simulink model "sampleModel7126_pp_1_1"  (R2018a)
settings: Solver=VariableStepAuto  StartTime=0.0  StopTime=10.0  RelTol=1e-3
undefined symbols (not defined in the file): DiscIntNeverNeededParam
libraries: simulink x367
(part 8 of 12)

== system sampleModel7126_pp_1_1/cfblk263/cfblk3 ==
  emi_1261 : Inport
  emi_1262 : Inport  Port=2
  Action Port : ActionPort  ActionType=then
  cfblk3 : simulink/Continuous/PID Controller (2DOF)  Controller=PID  TimeDomain=Discrete-time  SampleTime=-1  IntegratorMethod=Forward Euler  FilterMethod=Forward Euler  Form=Parallel  UseFilter=on  ControllerParametersSource=internal  P=1  I=1  D=0  N=100  b=1  c=1  InitialConditionSource=internal  InitialConditionForIntegrator=0  InitialConditionForFilter=0  ExternalReset=none  LimitOutput=off  UpperSaturationLimit=inf  LowerSaturationLimit=-inf  LinearizeAsGain=off  AntiWindupMode=none  Kb=1  TrackingMode=off  Kt=1  PParamMin=[]  PParamMax=[]  IParamMin=[]  IParamMax=[]  DParamMin=[]  DParamMax=[]  NParamMin=[]  NParamMax=[]  bParamMin=[]  bParamMax=[]  cParamMin=[]  cParamMax=[]  KbParamMin=[]  KbParamMax=[]  KtParamMin=[]  KtParamMax=[]  POutMin=[]  POutMax=[]  IOutMin=[]  IOutMax=[]  DOutMin=[]  DOutMax=[]  NOutMin=[]  NOutMax=[]  bOutMin=[]  bOutMax=[]  cOutMin=[]  cOutMax=[]  KbOutMin=[]  KbOutMax=[]  KtOutMin=[]  KtOutMax=[]  IntegratorOutMin=[]  IntegratorOutMax=[]  FilterOutMin=[]  FilterOutMax=[]  SumOutMin=[]  SumOutMax=[]  Sum1OutMin=[]  Sum1OutMax=[]  Sum2OutMin=[]  Sum2OutMax=[]  Sum3OutMin=[]  Sum3OutMax=[]  SumI1OutMin=[]  SumI1OutMax=[]  SumI2OutMin=[]  SumI2OutMax=[]  SumI3OutMin=[]  SumI3OutMax=[]  SumDOutMin=[]  SumDOutMax=[]  SaturationOutMin=[]  SaturationOutMax=[]  IntegratorContinuousStateAttributes=''  IntegratorStateMustResolveToSignalObject=off  IntegratorRTWStateStorageClass=Auto  FilterContinuousStateAttributes=''  FilterStateMustResolveToSignalObject=off  FilterRTWStateStorageClass=Auto  DifferentiatorICPrevScaledInput=0  DifferentiatorOutMin=[]  DifferentiatorOutMax=[]  FilterDiffOutCoefMin=[]  FilterDiffOutCoefMax=[]  SumDenOutMin=[]  SumDenOutMax=[]  SumNumOutMin=[]  SumNumOutMax=[]  ReciprocalOutMin=[]  ReciprocalOutMax=[]  DivideOutMin=[]  DivideOutMax=[]  TunerSelectOption=Transfer Function Based (PID Tuner App)
  emi_1263 : Outport
  wires:
  emi_1261/1 -> cfblk3/1
  emi_1262/1 -> cfblk3/2
  cfblk3/1 -> emi_1263/1

== system sampleModel7126_pp_1_1/cfblk263/cfblk4 ==
  emi_867 : Inport
  Action Port : ActionPort  ActionType=then
  cfblk4 : simulink/Discrete/Transfer Fcn Real Zero  ZeroZ=0.75  ICPrevInput=0.0  DoSatur=off
      settings: SourceProductName=Simulink  SourceProductBaseCode=SL
  emi_868 : Outport
  wires:
  emi_867/1 -> cfblk4/1
  cfblk4/1 -> emi_868/1

== system sampleModel7126_pp_1_1/cfblk263/cfblk8 ==
  emi_145 : Inport
  Action Port : ActionPort  ActionType=then
  cfblk8 : DiscreteFir
  emi_146 : Outport
  wires:
  emi_145/1 -> cfblk8/1
  cfblk8/1 -> emi_146/1

== system sampleModel7126_pp_1_1/cfblk263/cfblk9 ==
  emi_1276 : Inport
  Action Port : ActionPort  ActionType=then
  cfblk9 : DiscreteFir
  emi_1277 : Outport
  wires:
  emi_1276/1 -> cfblk9/1
  cfblk9/1 -> emi_1277/1

== system sampleModel7126_pp_1_1/cfblk263/emi_1264 ==
  Action Port : ActionPort  ActionType=else
  emi_1265 : Assertion

== system sampleModel7126_pp_1_1/cfblk263/emi_1278 ==
  Action Port : ActionPort  ActionType=else
  emi_1279 : Assertion

== system sampleModel7126_pp_1_1/cfblk263/emi_147 ==
  Action Port : ActionPort  ActionType=else
  emi_148 : Assertion

== system sampleModel7126_pp_1_1/cfblk263/emi_869 ==
  Action Port : ActionPort  ActionType=else
  emi_870 : Assertion

== system sampleModel7126_pp_1_1/cfblk264/cfblk10 ==
  emi_415 : Inport
  Action Port : ActionPort  ActionType=then
  cfblk10 : simulink/Discrete/Difference  ICPrevInput=0.0  OutMin=[]  OutMax=[]  OutDataTypeStr=double  OutputDataTypeScalingMode=double  OutDataType=fixdt(1, 16)  OutScaling=2^-10  DoSatur=off
  emi_416 : Outport
  wires:
  emi_415/1 -> cfblk10/1
  cfblk10/1 -> emi_416/1

== system sampleModel7126_pp_1_1/cfblk264/cfblk5 ==
  emi_995 : Inport
  Action Port : ActionPort  ActionType=then
  cfblk5 : DiscreteFir
  emi_996 : Outport
  wires:
  emi_995/1 -> cfblk5/1
  cfblk5/1 -> emi_996/1

== system sampleModel7126_pp_1_1/cfblk264/cfblk7 ==
  emi_230 : Inport
  emi_231 : Inport  Port=2
  Action Port : ActionPort  ActionType=then
  cfblk7 : Delay  DelayLengthSource=Input port
      settings: InputPortMap=u0,p1
  emi_232 : Outport
  wires:
  emi_230/1 -> cfblk7/1
  emi_231/1 -> cfblk7/2
  cfblk7/1 -> emi_232/1

== system sampleModel7126_pp_1_1/cfblk264/cfblk8 ==
  emi_1718 : Inport
  Action Port : ActionPort  ActionType=then
  cfblk8 : DiscreteTransferFcn
  emi_1719 : Outport
  wires:
  emi_1718/1 -> cfblk8/1
  cfblk8/1 -> emi_1719/1

== system sampleModel7126_pp_1_1/cfblk264/cfblk9 ==
  emi_1855 : Inport
  Action Port : ActionPort  ActionType=then
  cfblk9 : simulink/Continuous/PID Controller  Controller=PID  TimeDomain=Discrete-time  SampleTime=-1  IntegratorMethod=Forward Euler  FilterMethod=Forward Euler  Form=Parallel  UseFilter=on  ControllerParametersSource=internal  P=1  I=1  D=0  N=100  InitialConditionSource=internal  InitialConditionForIntegrator=0  InitialConditionForFilter=0  ExternalReset=none  LimitOutput=off  UpperSaturationLimit=inf  LowerSaturationLimit=-inf  LinearizeAsGain=off  AntiWindupMode=none  Kb=1  TrackingMode=off  Kt=1  PParamMin=[]  PParamMax=[]  IParamMin=[]  IParamMax=[]  DParamMin=[]  DParamMax=[]  NParamMin=[]  NParamMax=[]  KbParamMin=[]  KbParamMax=[]  KtParamMin=[]  KtParamMax=[]  POutMin=[]  POutMax=[]  IOutMin=[]  IOutMax=[]  DOutMin=[]  DOutMax=[]  NOutMin=[]  NOutMax=[]  KbOutMin=[]  KbOutMax=[]  KtOutMin=[]  KtOutMax=[]  IntegratorOutMin=[]  IntegratorOutMax=[]  FilterOutMin=[]  FilterOutMax=[]  SumOutMin=[]  SumOutMax=[]  SumI1OutMin=[]  SumI1OutMax=[]  SumI2OutMin=[]  SumI2OutMax=[]  SumI3OutMin=[]  SumI3OutMax=[]  SumDOutMin=[]  SumDOutMax=[]  SaturationOutMin=[]  SaturationOutMax=[]  IntegratorContinuousStateAttributes=''  IntegratorStateMustResolveToSignalObject=off  IntegratorRTWStateStorageClass=Auto  FilterContinuousStateAttributes=''  FilterStateMustResolveToSignalObject=off  FilterRTWStateStorageClass=Auto  DifferentiatorICPrevScaledInput=0  DifferentiatorOutMin=[]  DifferentiatorOutMax=[]  FilterDiffOutCoefMin=[]  FilterDiffOutCoefMax=[]  SumDenOutMin=[]  SumDenOutMax=[]  SumNumOutMin=[]  SumNumOutMax=[]  ReciprocalOutMin=[]  ReciprocalOutMax=[]  DivideOutMin=[]  DivideOutMax=[]  TunerSelectOption=Transfer Function Based (PID Tuner App)
  emi_1856 : Outport
  wires:
  emi_1855/1 -> cfblk9/1
  cfblk9/1 -> emi_1856/1

== system sampleModel7126_pp_1_1/cfblk264/emi_1720 ==
  Action Port : ActionPort  ActionType=else
  emi_1721 : Assertion

== system sampleModel7126_pp_1_1/cfblk264/emi_1857 ==
  Action Port : ActionPort  ActionType=else
  emi_1858 : Assertion

== system sampleModel7126_pp_1_1/cfblk264/emi_233 ==
  Action Port : ActionPort  ActionType=else
  emi_234 : Assertion

== system sampleModel7126_pp_1_1/cfblk264/emi_417 ==
  Action Port : ActionPort  ActionType=else
  emi_418 : Assertion

== system sampleModel7126_pp_1_1/cfblk264/emi_997 ==
  Action Port : ActionPort  ActionType=else
  emi_998 : Assertion

== system sampleModel7126_pp_1_1/cfblk265/cfblk10 ==
  cfblk1 : Inport
  cfblk11 : Inport  Port=2
  cfblk12 : Inport  Port=3
  cfblk13 : Inport  Port=4
  cfblk14 : Inport  Port=5
  Action Port : ActionPort  ActionType=else
  cfblk10 : DiscreteStateSpace  SampleTime=-1
  cfblk3 : Delay
  cfblk4 : DiscreteFir
  cfblk5 : simulink/Discrete/Transfer Fcn Lead or Lag  PoleZ=0.95  ZeroZ=0.75  ICPrevOutput=0.0  ICPrevInput=0.0  DoSatur=off
      settings: SourceProductName=Simulink  SourceProductBaseCode=SL
  cfblk6 : Subsystem  TreatAsAtomicUnit=on
  cfblk7 : DiscreteZeroPole  Poles=[0 0.5]  Gain=1  SampleTime=-1
  cfblk8 : DiscreteZeroPole  Poles=[0 0.5]  Gain=1  SampleTime=-1
  cfblk9 : simulink/Discrete/Difference  ICPrevInput=0.0  OutMin=[]  OutMax=[]  OutDataTypeStr=double  OutputDataTypeScalingMode=double  OutDataType=fixdt(1, 16)  OutScaling=2^-10  DoSatur=off
  cyemi_{554..561} (8 alike) : DataTypeConversion  OutDataTypeStr=double
  emi_933 : Subsystem  TreatAsAtomicUnit=on
  emi_935 : If  IfExpression=0 <= u1  SampleTime=[1 0]
  emi_936 : DataTypeConversion  OutDataTypeStr=double
  cfblk2 : Outport
  cfblk15 : Outport  Port=2
  wires:
  cfblk3/1 -> cfblk15/1
  cfblk11/1 -> cfblk2/1
  cyemi_554/1 -> cfblk10/1
  cfblk13/1 -> cyemi_554/1
  cyemi_555/1 -> cfblk3/1
  cfblk8/1 -> cyemi_555/1
  cyemi_556/1 -> cfblk4/1
  cfblk14/1 -> cyemi_556/1
  cyemi_557/1 -> cfblk5/1
  cfblk4/1 -> cyemi_557/1
  cfblk12/1 -> cyemi_558/1
  cyemi_559/1 -> cfblk7/1
  cfblk1/1 -> cyemi_559/1
  cyemi_560/1 -> cfblk8/1
  cyemi_561/1 -> cfblk9/1
  cfblk7/1 -> cyemi_561/1, emi_936/1
  cyemi_558/1 -> cfblk6/1(emi_931)
  cfblk6/1(emi_932) -> cyemi_560/1
  emi_935/1 -> cfblk6/Action
  emi_935/2 -> emi_933/Action
  emi_936/1 -> emi_935/1

== system sampleModel7126_pp_1_1/cfblk265/cfblk12 ==
  emi_287 : Inport
  Action Port : ActionPort  ActionType=then
  cfblk12 : Delay
  emi_288 : Outport
  wires:
  emi_287/1 -> cfblk12/1
  cfblk12/1 -> emi_288/1

== system sampleModel7126_pp_1_1/cfblk265/cfblk3 ==
  emi_1305 : Inport
  emi_1306 : Inport  Port=2
  Action Port : ActionPort  ActionType=then
  cfblk3 : Delay  DelayLengthSource=Input port
      settings: InputPortMap=u0,p1
  emi_1307 : Outport
  wires:
  emi_1305/1 -> cfblk3/1
  emi_1306/1 -> cfblk3/2
  cfblk3/1 -> emi_1307/1

== system sampleModel7126_pp_1_1/cfblk265/cfblk9 ==
  cfblk1 : Inport
  cfblk10 : Inport  Port=2
  cfblk11 : Inport  Port=3
  Action Port : ActionPort  ActionType=then
  cfblk3 : DiscreteIntegrator  SampleTime=-1  OutDataTypeStr=double  ICPrevOutput=DiscIntNeverNeededParam  ICPrevScaledInput=DiscIntNeverNeededParam
  cfblk4 : simulink/Continuous/PID Controller  Controller=PID  TimeDomain=Discrete-time  SampleTime=-1  IntegratorMethod=Forward Euler  FilterMethod=Forward Euler  Form=Parallel  UseFilter=on  ControllerParametersSource=internal  P=1  I=1  D=0  N=100  InitialConditionSource=internal  InitialConditionForIntegrator=0  InitialConditionForFilter=0  ExternalReset=none  LimitOutput=off  UpperSaturationLimit=inf  LowerSaturationLimit=-inf  LinearizeAsGain=off  AntiWindupMode=none  Kb=1  TrackingMode=off  Kt=1  PParamMin=[]  PParamMax=[]  IParamMin=[]  IParamMax=[]  DParamMin=[]  DParamMax=[]  NParamMin=[]  NParamMax=[]  KbParamMin=[]  KbParamMax=[]  KtParamMin=[]  KtParamMax=[]  POutMin=[]  POutMax=[]  IOutMin=[]  IOutMax=[]  DOutMin=[]  DOutMax=[]  NOutMin=[]  NOutMax=[]  KbOutMin=[]  KbOutMax=[]  KtOutMin=[]  KtOutMax=[]  IntegratorOutMin=[]  IntegratorOutMax=[]  FilterOutMin=[]  FilterOutMax=[]  SumOutMin=[]  SumOutMax=[]  SumI1OutMin=[]  SumI1OutMax=[]  SumI2OutMin=[]  SumI2OutMax=[]  SumI3OutMin=[]  SumI3OutMax=[]  SumDOutMin=[]  SumDOutMax=[]  SaturationOutMin=[]  SaturationOutMax=[]  IntegratorContinuousStateAttributes=''  IntegratorStateMustResolveToSignalObject=off  IntegratorRTWStateStorageClass=Auto  FilterContinuousStateAttributes=''  FilterStateMustResolveToSignalObject=off  FilterRTWStateStorageClass=Auto  DifferentiatorICPrevScaledInput=0  DifferentiatorOutMin=[]  DifferentiatorOutMax=[]  FilterDiffOutCoefMin=[]  FilterDiffOutCoefMax=[]  SumDenOutMin=[]  SumDenOutMax=[]  SumNumOutMin=[]  SumNumOutMax=[]  ReciprocalOutMin=[]  ReciprocalOutMax=[]  DivideOutMin=[]  DivideOutMax=[]  TunerSelectOption=Transfer Function Based (PID Tuner App)
  cfblk5 : simulink/Continuous/PID Controller (2DOF)  Controller=PID  TimeDomain=Discrete-time  SampleTime=-1  IntegratorMethod=Forward Euler  FilterMethod=Forward Euler  Form=Parallel  UseFilter=on  ControllerParametersSource=internal  P=1  I=1  D=0  N=100  b=1  c=1  InitialConditionSource=internal  InitialConditionForIntegrator=0  InitialConditionForFilter=0  ExternalReset=none  LimitOutput=off  UpperSaturationLimit=inf  LowerSaturationLimit=-inf  LinearizeAsGain=off  AntiWindupMode=none  Kb=1  TrackingMode=off  Kt=1  PParamMin=[]  PParamMax=[]  IParamMin=[]  IParamMax=[]  DParamMin=[]  DParamMax=[]  NParamMin=[]  NParamMax=[]  bParamMin=[]  bParamMax=[]  cParamMin=[]  cParamMax=[]  KbParamMin=[]  KbParamMax=[]  KtParamMin=[]  KtParamMax=[]  POutMin=[]  POutMax=[]  IOutMin=[]  IOutMax=[]  DOutMin=[]  DOutMax=[]  NOutMin=[]  NOutMax=[]  bOutMin=[]  bOutMax=[]  cOutMin=[]  cOutMax=[]  KbOutMin=[]  KbOutMax=[]  KtOutMin=[]  KtOutMax=[]  IntegratorOutMin=[]  IntegratorOutMax=[]  FilterOutMin=[]  FilterOutMax=[]  SumOutMin=[]  SumOutMax=[]  Sum1OutMin=[]  Sum1OutMax=[]  Sum2OutMin=[]  Sum2OutMax=[]  Sum3OutMin=[]  Sum3OutMax=[]  SumI1OutMin=[]  SumI1OutMax=[]  SumI2OutMin=[]  SumI2OutMax=[]  SumI3OutMin=[]  SumI3OutMax=[]  SumDOutMin=[]  SumDOutMax=[]  SaturationOutMin=[]  SaturationOutMax=[]  IntegratorContinuousStateAttributes=''  IntegratorStateMustResolveToSignalObject=off  IntegratorRTWStateStorageClass=Auto  FilterContinuousStateAttributes=''  FilterStateMustResolveToSignalObject=off  FilterRTWStateStorageClass=Auto  DifferentiatorICPrevScaledInput=0  DifferentiatorOutMin=[]  DifferentiatorOutMax=[]  FilterDiffOutCoefMin=[]  FilterDiffOutCoefMax=[]  SumDenOutMin=[]  SumDenOutMax=[]  SumNumOutMin=[]  SumNumOutMax=[]  ReciprocalOutMin=[]  ReciprocalOutMax=[]  DivideOutMin=[]  DivideOutMax=[]  TunerSelectOption=Transfer Function Based (PID Tuner App)
  cfblk6 : simulink/Discrete/Transfer Fcn Lead or Lag  PoleZ=0.95  ZeroZ=0.75  ICPrevOutput=0.0  ICPrevInput=0.0  DoSatur=off
      settings: SourceProductName=Simulink  SourceProductBaseCode=SL
  cfblk7 : DiscreteFir
  cfblk8 : DiscreteFir
  cfblk9 : simulink/Continuous/PID Controller (2DOF)  Controller=PID  TimeDomain=Discrete-time  SampleTime=-1  IntegratorMethod=Forward Euler  FilterMethod=Forward Euler  Form=Parallel  UseFilter=on  ControllerParametersSource=internal  P=1  I=1  D=0  N=100  b=1  c=1  InitialConditionSource=internal  InitialConditionForIntegrator=0  InitialConditionForFilter=0  ExternalReset=none  LimitOutput=off  UpperSaturationLimit=inf  LowerSaturationLimit=-inf  LinearizeAsGain=off  AntiWindupMode=none  Kb=1  TrackingMode=off  Kt=1  PParamMin=[]  PParamMax=[]  IParamMin=[]  IParamMax=[]  DParamMin=[]  DParamMax=[]  NParamMin=[]  NParamMax=[]  bParamMin=[]  bParamMax=[]  cParamMin=[]  cParamMax=[]  KbParamMin=[]  KbParamMax=[]  KtParamMin=[]  KtParamMax=[]  POutMin=[]  POutMax=[]  IOutMin=[]  IOutMax=[]  DOutMin=[]  DOutMax=[]  NOutMin=[]  NOutMax=[]  bOutMin=[]  bOutMax=[]  cOutMin=[]  cOutMax=[]  KbOutMin=[]  KbOutMax=[]  KtOutMin=[]  KtOutMax=[]  IntegratorOutMin=[]  IntegratorOutMax=[]  FilterOutMin=[]  FilterOutMax=[]  SumOutMin=[]  SumOutMax=[]  Sum1OutMin=[]  Sum1OutMax=[]  Sum2OutMin=[]  Sum2OutMax=[]  Sum3OutMin=[]  Sum3OutMax=[]  SumI1OutMin=[]  SumI1OutMax=[]  SumI2OutMin=[]  SumI2OutMax=[]  SumI3OutMin=[]  SumI3OutMax=[]  SumDOutMin=[]  SumDOutMax=[]  SaturationOutMin=[]  SaturationOutMax=[]  IntegratorContinuousStateAttributes=''  IntegratorStateMustResolveToSignalObject=off  IntegratorRTWStateStorageClass=Auto  FilterContinuousStateAttributes=''  FilterStateMustResolveToSignalObject=off  FilterRTWStateStorageClass=Auto  DifferentiatorICPrevScaledInput=0  DifferentiatorOutMin=[]  DifferentiatorOutMax=[]  FilterDiffOutCoefMin=[]  FilterDiffOutCoefMax=[]  SumDenOutMin=[]  SumDenOutMax=[]  SumNumOutMin=[]  SumNumOutMax=[]  ReciprocalOutMin=[]  ReciprocalOutMax=[]  DivideOutMin=[]  DivideOutMax=[]  TunerSelectOption=Transfer Function Based (PID Tuner App)
  cyemi_{580..588} (9 alike) : DataTypeConversion  OutDataTypeStr=double
  cfblk2 : Outport
  wires:
  cfblk6/1 -> cfblk2/1
  cyemi_580/1 -> cfblk3/1
  cfblk1/1 -> cyemi_580/1
  cyemi_581/1 -> cfblk4/1
  cfblk9/1 -> cyemi_581/1
  cyemi_582/1 -> cfblk5/1
  cfblk10/1 -> cyemi_582/1
  cyemi_583/1 -> cfblk5/2
  cfblk7/1 -> cyemi_583/1
  cyemi_584/1 -> cfblk6/1
  cfblk5/1 -> cyemi_584/1
  cyemi_585/1 -> cfblk7/1
  cfblk4/1 -> cyemi_585/1
  cyemi_586/1 -> cfblk8/1
  cfblk3/1 -> cyemi_586/1
  cyemi_587/1 -> cfblk9/1
  cfblk8/1 -> cyemi_587/1
  cyemi_588/1 -> cfblk9/2
  cfblk11/1 -> cyemi_588/1

== system sampleModel7126_pp_1_1/cfblk265/emi_1308 ==
  Action Port : ActionPort  ActionType=else
  emi_1309 : Assertion

== system sampleModel7126_pp_1_1/cfblk265/emi_289 ==
  Action Port : ActionPort  ActionType=else
  emi_290 : Assertion

== system sampleModel7126_pp_1_1/cfblk266/cfblk10 ==
  cfblk1 : Inport
  Action Port : ActionPort  ActionType=else
  cfblk3 : Subsystem  TreatAsAtomicUnit=on
  cfblk4 : Subsystem  TreatAsAtomicUnit=on
  cfblk5 : Subsystem  TreatAsAtomicUnit=on
  cfblk6 : simulink/Discrete/Transfer Fcn Lead or Lag  PoleZ=0.95  ZeroZ=0.75  ICPrevOutput=0.0  ICPrevInput=0.0  DoSatur=off
      settings: SourceProductName=Simulink  SourceProductBaseCode=SL
  cfblk8 : Subsystem  TreatAsAtomicUnit=on
  cyemi_{591..597} (7 alike) : DataTypeConversion  OutDataTypeStr=double
  emi_1880 : Subsystem  TreatAsAtomicUnit=on
  emi_1882 : If  IfExpression=0 <= u1  SampleTime=[1 0]
  emi_{271,526,617,1883} (4 alike) : DataTypeConversion  OutDataTypeStr=double
  emi_268 : Subsystem  TreatAsAtomicUnit=on
  emi_270 : If  IfExpression=0 <= u1
  emi_523 : Subsystem  TreatAsAtomicUnit=on
  emi_525 : If  IfExpression=0 <= u1  SampleTime=[1 0]
  emi_614 : Subsystem  TreatAsAtomicUnit=on
  emi_616 : If  IfExpression=0 <= u1  SampleTime=[1 0]
  cfblk2 : Outport
  cfblk7 : Outport  Port=2
  wires:
  cfblk6/1 -> cyemi_591/1, cyemi_594/1
  cfblk1/1 -> cyemi_593/1
  cyemi_596/1 -> cfblk6/1
  cyemi_591/1 -> cfblk3/1(emi_266)
  cfblk3/1(emi_267) -> cyemi_597/1
  emi_270/1 -> cfblk3/Action
  emi_270/2 -> emi_268/Action
  emi_271/1 -> emi_270/1
  cyemi_594/1 -> cfblk5/1(emi_520)
  cyemi_595/1 -> cfblk5/2(emi_521)
  cfblk5/1(emi_522) -> cfblk7/1, cfblk2/1, emi_617/1, emi_1883/1
  emi_525/1 -> cfblk5/Action
  emi_525/2 -> emi_523/Action
  emi_526/1 -> emi_525/1
  cyemi_597/1 -> cfblk8/1(emi_612)
  cfblk8/1(emi_613) -> emi_526/1, emi_271/1, cyemi_592/1
  emi_616/1 -> cfblk8/Action
  emi_616/2 -> emi_614/Action
  emi_617/1 -> emi_616/1
  cyemi_592/1 -> cfblk4/1(emi_1877)
  cyemi_593/1 -> cfblk4/2(emi_1878)
  cfblk4/1(emi_1879) -> cyemi_596/1, cyemi_595/1
  emi_1882/1 -> cfblk4/Action
  emi_1882/2 -> emi_1880/Action
  emi_1883/1 -> emi_1882/1

== system sampleModel7126_pp_1_1/cfblk266/cfblk12 ==
  emi_924 : Inport
  Action Port : ActionPort  ActionType=then
  cfblk12 : Delay
  emi_925 : Outport
  wires:
  emi_924/1 -> cfblk12/1
  cfblk12/1 -> emi_925/1

== system sampleModel7126_pp_1_1/cfblk266/cfblk14 ==
  emi_1224 : Inport
  Action Port : ActionPort  ActionType=then
  cfblk14 : Delay
  emi_1225 : Outport
  wires:
  emi_1224/1 -> cfblk14/1
  cfblk14/1 -> emi_1225/1

== system sampleModel7126_pp_1_1/cfblk266/cfblk3 ==
  emi_1469 : Inport
  Action Port : ActionPort  ActionType=then
  cfblk3 : UnitDelay  SampleTime=-1
  emi_1470 : Outport
  wires:
  emi_1469/1 -> cfblk3/1
  cfblk3/1 -> emi_1470/1

== system sampleModel7126_pp_1_1/cfblk266/cfblk9 ==
  cfblk1 : Inport
  cfblk6 : Inport  Port=2
  cfblk7 : Inport  Port=3
  Action Port : ActionPort  ActionType=then
  cfblk3 : simulink/Discrete/Difference  ICPrevInput=0.0  OutMin=[]  OutMax=[]  OutDataTypeStr=double  OutputDataTypeScalingMode=double  OutDataType=fixdt(1, 16)  OutScaling=2^-10  DoSatur=off
  cfblk4 : simulink/Discrete/Transfer Fcn Lead or Lag  PoleZ=0.95  ZeroZ=0.75  ICPrevOutput=0.0  ICPrevInput=0.0  DoSatur=off
      settings: SourceProductName=Simulink  SourceProductBaseCode=SL
  cfblk5 : DiscreteIntegrator  SampleTime=-1  OutDataTypeStr=double  ICPrevOutput=DiscIntNeverNeededParam  ICPrevScaledInput=DiscIntNeverNeededParam
  cyemi_612 : DataTypeConversion  OutDataTypeStr=double
  cyemi_613 : DataTypeConversion  OutDataTypeStr=double
  cyemi_614 : DataTypeConversion  OutDataTypeStr=double
  cfblk2 : Outport
  cfblk8 : Outport  Port=2
  wires:
  cfblk5/1 -> cfblk8/1
  cfblk3/1 -> cfblk2/1
  cyemi_612/1 -> cfblk3/1
  cfblk7/1 -> cyemi_612/1
  cyemi_613/1 -> cfblk4/1
  cfblk6/1 -> cyemi_613/1
  cyemi_614/1 -> cfblk5/1
  cfblk1/1 -> cyemi_614/1

== system sampleModel7126_pp_1_1/cfblk266/emi_1226 ==
  Action Port : ActionPort  ActionType=else
  emi_1227 : Assertion

== system sampleModel7126_pp_1_1/cfblk266/emi_1471 ==
  Action Port : ActionPort  ActionType=else
  emi_1472 : Assertion

== system sampleModel7126_pp_1_1/cfblk266/emi_926 ==
  Action Port : ActionPort  ActionType=else
  emi_927 : Assertion

== system sampleModel7126_pp_1_1/cfblk267/cfblk10 ==
  emi_2180 : Inport
  Action Port : ActionPort  ActionType=then
  cfblk10 : DiscreteFilter
  emi_2181 : Outport
  wires:
  emi_2180/1 -> cfblk10/1
  cfblk10/1 -> emi_2181/1

== system sampleModel7126_pp_1_1/cfblk267/cfblk11 ==
  emi_245 : Inport
  Action Port : ActionPort  ActionType=then
  cfblk11 : Delay
  emi_246 : Outport
  wires:
  emi_245/1 -> cfblk11/1
  cfblk11/1 -> emi_246/1

== system sampleModel7126_pp_1_1/cfblk267/cfblk3 ==
  emi_528 : Inport
  Action Port : ActionPort  ActionType=then
  cfblk3 : DiscreteFir
  emi_529 : Outport
  wires:
  emi_528/1 -> cfblk3/1
  cfblk3/1 -> emi_529/1

== system sampleModel7126_pp_1_1/cfblk267/cfblk4 ==
  emi_1334 : Inport
  Action Port : ActionPort  ActionType=then
  cfblk4 : UnitDelay  SampleTime=-1
  emi_1335 : Outport
  wires:
  emi_1334/1 -> cfblk4/1
  cfblk4/1 -> emi_1335/1

== system sampleModel7126_pp_1_1/cfblk267/cfblk5 ==
  emi_1298 : Inport
  Action Port : ActionPort  ActionType=then
  cfblk5 : simulink/Continuous/PID Controller  Controller=PID  TimeDomain=Discrete-time  SampleTime=-1  IntegratorMethod=Forward Euler  FilterMethod=Forward Euler  Form=Parallel  UseFilter=on  ControllerParametersSource=internal  P=1  I=1  D=0  N=100  InitialConditionSource=internal  InitialConditionForIntegrator=0  InitialConditionForFilter=0  ExternalReset=none  LimitOutput=off  UpperSaturationLimit=inf  LowerSaturationLimit=-inf  LinearizeAsGain=off  AntiWindupMode=none  Kb=1  TrackingMode=off  Kt=1  PParamMin=[]  PParamMax=[]  IParamMin=[]  IParamMax=[]  DParamMin=[]  DParamMax=[]  NParamMin=[]  NParamMax=[]  KbParamMin=[]  KbParamMax=[]  KtParamMin=[]  KtParamMax=[]  POutMin=[]  POutMax=[]  IOutMin=[]  IOutMax=[]  DOutMin=[]  DOutMax=[]  NOutMin=[]  NOutMax=[]  KbOutMin=[]  KbOutMax=[]  KtOutMin=[]  KtOutMax=[]  IntegratorOutMin=[]  IntegratorOutMax=[]  FilterOutMin=[]  FilterOutMax=[]  SumOutMin=[]  SumOutMax=[]  SumI1OutMin=[]  SumI1OutMax=[]  SumI2OutMin=[]  SumI2OutMax=[]  SumI3OutMin=[]  SumI3OutMax=[]  SumDOutMin=[]  SumDOutMax=[]  SaturationOutMin=[]  SaturationOutMax=[]  IntegratorContinuousStateAttributes=''  IntegratorStateMustResolveToSignalObject=off  IntegratorRTWStateStorageClass=Auto  FilterContinuousStateAttributes=''  FilterStateMustResolveToSignalObject=off  FilterRTWStateStorageClass=Auto  DifferentiatorICPrevScaledInput=0  DifferentiatorOutMin=[]  DifferentiatorOutMax=[]  FilterDiffOutCoefMin=[]  FilterDiffOutCoefMax=[]  SumDenOutMin=[]  SumDenOutMax=[]  SumNumOutMin=[]  SumNumOutMax=[]  ReciprocalOutMin=[]  ReciprocalOutMax=[]  DivideOutMin=[]  DivideOutMax=[]  TunerSelectOption=Transfer Function Based (PID Tuner App)
  emi_1299 : Outport
  wires:
  emi_1298/1 -> cfblk5/1
  cfblk5/1 -> emi_1299/1

== system sampleModel7126_pp_1_1/cfblk267/cfblk7 ==
  emi_960 : Inport
  Action Port : ActionPort  ActionType=then
  cfblk7 : DiscreteStateSpace  SampleTime=-1
  emi_961 : Outport
  wires:
  emi_960/1 -> cfblk7/1
  cfblk7/1 -> emi_961/1

== system sampleModel7126_pp_1_1/cfblk267/cfblk8 ==
  emi_1117 : Inport
  Action Port : ActionPort  ActionType=then
  cfblk8 : DiscreteZeroPole  Poles=[0 0.5]  Gain=1  SampleTime=-1
  emi_1118 : Outport
  wires:
  emi_1117/1 -> cfblk8/1
  cfblk8/1 -> emi_1118/1

== system sampleModel7126_pp_1_1/cfblk267/emi_1119 ==
  Action Port : ActionPort  ActionType=else
  emi_1120 : Assertion

== system sampleModel7126_pp_1_1/cfblk267/emi_1300 ==
  Action Port : ActionPort  ActionType=else
  emi_1301 : Assertion

== system sampleModel7126_pp_1_1/cfblk267/emi_1336 ==
  Action Port : ActionPort  ActionType=else
  emi_1337 : Assertion

== system sampleModel7126_pp_1_1/cfblk267/emi_2182 ==
  Action Port : ActionPort  ActionType=else
  emi_2183 : Assertion

== system sampleModel7126_pp_1_1/cfblk267/emi_247 ==
  Action Port : ActionPort  ActionType=else
  emi_248 : Assertion

== system sampleModel7126_pp_1_1/cfblk267/emi_530 ==
  Action Port : ActionPort  ActionType=else
  emi_531 : Assertion

== system sampleModel7126_pp_1_1/cfblk267/emi_962 ==
  Action Port : ActionPort  ActionType=else
  emi_963 : Assertion

== system sampleModel7126_pp_1_1/cfblk268/cfblk3 ==
  emi_640 : Inport
  Action Port : ActionPort  ActionType=then
  cfblk3 : DiscreteStateSpace  SampleTime=-1
  emi_641 : Outport
  wires:
  emi_640/1 -> cfblk3/1
  cfblk3/1 -> emi_641/1

== system sampleModel7126_pp_1_1/cfblk268/cfblk5 ==
  emi_1689 : Inport
  Action Port : ActionPort  ActionType=then
  cfblk5 : simulink/Discrete/Transfer Fcn Real Zero  ZeroZ=0.75  ICPrevInput=0.0  DoSatur=off
      settings: SourceProductName=Simulink  SourceProductBaseCode=SL
  emi_1690 : Outport
  wires:
  emi_1689/1 -> cfblk5/1
  cfblk5/1 -> emi_1690/1

== system sampleModel7126_pp_1_1/cfblk268/cfblk8 ==
  emi_1562 : Inport
  Action Port : ActionPort  ActionType=then
  cfblk8 : simulink/Discrete/Transfer Fcn Lead or Lag  PoleZ=0.95  ZeroZ=0.75  ICPrevOutput=0.0  ICPrevInput=0.0  DoSatur=off
      settings: SourceProductName=Simulink  SourceProductBaseCode=SL
  emi_1563 : Outport
  wires:
  emi_1562/1 -> cfblk8/1
  cfblk8/1 -> emi_1563/1

== system sampleModel7126_pp_1_1/cfblk268/emi_1564 ==
  Action Port : ActionPort  ActionType=else
  emi_1565 : Assertion

== system sampleModel7126_pp_1_1/cfblk268/emi_1691 ==
  Action Port : ActionPort  ActionType=else
  emi_1692 : Assertion

== system sampleModel7126_pp_1_1/cfblk268/emi_642 ==
  Action Port : ActionPort  ActionType=else
  emi_643 : Assertion

== system sampleModel7126_pp_1_1/cfblk269/cfblk14 ==
  emi_1740 : Inport
  Action Port : ActionPort  ActionType=then
  cfblk14 : Delay
  emi_1741 : Outport
  wires:
  emi_1740/1 -> cfblk14/1
  cfblk14/1 -> emi_1741/1

== system sampleModel7126_pp_1_1/cfblk269/cfblk3 ==
  emi_1777 : Inport
  Action Port : ActionPort  ActionType=then
  cfblk3 : DiscreteIntegrator  SampleTime=-1  OutDataTypeStr=double  ICPrevOutput=DiscIntNeverNeededParam  ICPrevScaledInput=DiscIntNeverNeededParam
  emi_1778 : Outport
  wires:
  emi_1777/1 -> cfblk3/1
  cfblk3/1 -> emi_1778/1

== system sampleModel7126_pp_1_1/cfblk269/cfblk4 ==
  emi_489 : Inport
  emi_490 : Inport  Port=2
  Action Port : ActionPort  ActionType=then
  cfblk4 : Delay  ShowEnablePort=on
      settings: InputPortMap=u0,e6
  emi_491 : Outport
  wires:
  emi_489/1 -> cfblk4/1
  emi_490/1 -> cfblk4/2
  cfblk4/1 -> emi_491/1

== system sampleModel7126_pp_1_1/cfblk269/cfblk8 ==
  cfblk1 : Inport
  cfblk12 : Inport  Port=2
  cfblk13 : Inport  Port=3
  Action Port : ActionPort  ActionType=then
  cfblk10 : Delay  ShowEnablePort=on
      settings: InputPortMap=u0,e6
  cfblk11 : Subsystem  TreatAsAtomicUnit=on
  cfblk15 : Delay
  cfblk3 : simulink/Continuous/PID Controller  Controller=PID  TimeDomain=Discrete-time  SampleTime=-1  IntegratorMethod=Forward Euler  FilterMethod=Forward Euler  Form=Parallel  UseFilter=on  ControllerParametersSource=internal  P=1  I=1  D=0  N=100  InitialConditionSource=internal  InitialConditionForIntegrator=0  InitialConditionForFilter=0  ExternalReset=none  LimitOutput=off  UpperSaturationLimit=inf  LowerSaturationLimit=-inf  LinearizeAsGain=off  AntiWindupMode=none  Kb=1  TrackingMode=off  Kt=1  PParamMin=[]  PParamMax=[]  IParamMin=[]  IParamMax=[]  DParamMin=[]  DParamMax=[]  NParamMin=[]  NParamMax=[]  KbParamMin=[]  KbParamMax=[]  KtParamMin=[]  KtParamMax=[]  POutMin=[]  POutMax=[]  IOutMin=[]  IOutMax=[]  DOutMin=[]  DOutMax=[]  NOutMin=[]  NOutMax=[]  KbOutMin=[]  KbOutMax=[]  KtOutMin=[]  KtOutMax=[]  IntegratorOutMin=[]  IntegratorOutMax=[]  FilterOutMin=[]  FilterOutMax=[]  SumOutMin=[]  SumOutMax=[]  SumI1OutMin=[]  SumI1OutMax=[]  SumI2OutMin=[]  SumI2OutMax=[]  SumI3OutMin=[]  SumI3OutMax=[]  SumDOutMin=[]  SumDOutMax=[]  SaturationOutMin=[]  SaturationOutMax=[]  IntegratorContinuousStateAttributes=''  IntegratorStateMustResolveToSignalObject=off  IntegratorRTWStateStorageClass=Auto  FilterContinuousStateAttributes=''  FilterStateMustResolveToSignalObject=off  FilterRTWStateStorageClass=Auto  DifferentiatorICPrevScaledInput=0  DifferentiatorOutMin=[]  DifferentiatorOutMax=[]  FilterDiffOutCoefMin=[]  FilterDiffOutCoefMax=[]  SumDenOutMin=[]  SumDenOutMax=[]  SumNumOutMin=[]  SumNumOutMax=[]  ReciprocalOutMin=[]  ReciprocalOutMax=[]  DivideOutMin=[]  DivideOutMax=[]  TunerSelectOption=Transfer Function Based (PID Tuner App)
  cfblk4 : UnitDelay  SampleTime=-1
  cfblk5 : DiscreteIntegrator  SampleTime=-1  OutDataTypeStr=double  ICPrevOutput=DiscIntNeverNeededParam  ICPrevScaledInput=DiscIntNeverNeededParam
  cfblk6 : simulink/Discrete/Tapped Delay  vinit=0.0  samptime=-1  NumDelays=1  DelayOrder=Oldest  includeCurrent=off
  cfblk7 : Subsystem  TreatAsAtomicUnit=on
  cfblk8 : DiscreteZeroPole  Poles=[0 0.5]  Gain=1  SampleTime=-1
  cfblk9 : DiscreteStateSpace  SampleTime=-1
  cyemi_{653..663} (11 alike) : DataTypeConversion  OutDataTypeStr=double
  emi_2075 : Subsystem  TreatAsAtomicUnit=on
  emi_2077 : If  IfExpression=Inf <= u1  SampleTime=[1 0]
  emi_2078 : DataTypeConversion  OutDataTypeStr=double
  emi_955 : Subsystem  TreatAsAtomicUnit=on
  emi_957 : If  IfExpression=Inf <= u1  SampleTime=[1 0]
  emi_958 : DataTypeConversion  OutDataTypeStr=double
  cfblk2 : Outport
  cfblk14 : Outport  Port=2
  wires:
  cfblk8/1 -> cfblk14/1, emi_958/1
  cfblk1/1 -> cfblk2/1
  cyemi_653/1 -> cfblk10/1
  cfblk13/1 -> cyemi_653/1
  cyemi_654/1 -> cfblk10/2
  cfblk3/1 -> cyemi_655/1
  cyemi_656/1 -> cfblk15/1
  cfblk5/1 -> cyemi_656/1
  cyemi_657/1 -> cfblk3/1
  cfblk9/1 -> cyemi_657/1
  cyemi_658/1 -> cfblk4/1
  cfblk15/1 -> cyemi_658/1
  cyemi_659/1 -> cfblk5/1
  cfblk4/1 -> cyemi_659/1, emi_2078/1
  cyemi_660/1 -> cfblk6/1
  cfblk12/1 -> cyemi_660/1
  cyemi_662/1 -> cfblk8/1
  cfblk10/1 -> cyemi_662/1
  cyemi_663/1 -> cfblk9/1
  cfblk6/1 -> cyemi_663/1
  cyemi_655/1 -> cfblk11/1(emi_953)
  cfblk11/1(emi_954) -> cyemi_661/1
  emi_957/1 -> cfblk11/Action
  emi_957/2 -> emi_955/Action
  emi_958/1 -> emi_957/1
  cyemi_661/1 -> cfblk7/1(emi_2073)
  cfblk7/1(emi_2074) -> cyemi_654/1
  emi_2077/1 -> cfblk7/Action
  emi_2077/2 -> emi_2075/Action
  emi_2078/1 -> emi_2077/1

== system sampleModel7126_pp_1_1/cfblk269/cfblk9 ==
  cfblk1 : Inport
  cfblk8 : Inport  Port=2
  cfblk9 : Inport  Port=3
  Action Port : ActionPort  ActionType=else
  cfblk3 : DiscreteStateSpace  SampleTime=-1
  cfblk4 : DiscreteFilter
  cfblk5 : Subsystem  TreatAsAtomicUnit=on
  cfblk6 : Subsystem  TreatAsAtomicUnit=on
  cfblk7 : DiscreteStateSpace  SampleTime=-1
  cyemi_{667..672} (6 alike) : DataTypeConversion  OutDataTypeStr=double
  emi_1198 : Subsystem  TreatAsAtomicUnit=on
  emi_1200 : If  IfExpression=Inf <= u1  SampleTime=[1 0]
  emi_1201 : DataTypeConversion  OutDataTypeStr=double
  emi_275 : Subsystem  TreatAsAtomicUnit=on
  emi_277 : If  IfExpression=Inf <= u1  SampleTime=[1 0]
  emi_278 : DataTypeConversion  OutDataTypeStr=double
  cfblk2 : Outport
  cfblk10 : Outport  Port=2
  cfblk11 : Outport  Port=3
  cfblk12 : Outport  Port=4
  cfblk13 : Outport  Port=5
  wires:
  cfblk1/1 -> cyemi_668/1, cyemi_669/1
  cfblk3/1 -> cfblk10/1, cyemi_670/1, emi_1201/1
  cfblk9/1 -> cfblk13/1
  cfblk4/1 -> cfblk11/1, cyemi_667/1
  cfblk7/1 -> cfblk2/1, emi_278/1
  cyemi_667/1 -> cfblk3/1
  cyemi_668/1 -> cfblk4/1
  cyemi_672/1 -> cfblk7/1
  cfblk8/1 -> cyemi_672/1
  cyemi_671/1 -> cfblk6/1(emi_273)
  cfblk6/1(emi_274) -> cfblk12/1
  emi_277/1 -> cfblk6/Action
  emi_277/2 -> emi_275/Action
  emi_278/1 -> emi_277/1
  cyemi_669/1 -> cfblk5/1(emi_1195)
  cyemi_670/1 -> cfblk5/2(emi_1196)
  cfblk5/1(emi_1197) -> cyemi_671/1
  emi_1200/1 -> cfblk5/Action
  emi_1200/2 -> emi_1198/Action
  emi_1201/1 -> emi_1200/1

== system sampleModel7126_pp_1_1/cfblk269/emi_1742 ==
  Action Port : ActionPort  ActionType=else
  emi_1743 : Assertion

== system sampleModel7126_pp_1_1/cfblk269/emi_1779 ==
  Action Port : ActionPort  ActionType=else
  emi_1780 : Assertion

== system sampleModel7126_pp_1_1/cfblk269/emi_492 ==
  Action Port : ActionPort  ActionType=else
  emi_493 : Assertion

== system sampleModel7126_pp_1_1/cfblk270/cfblk11 ==
  emi_2045 : Inport
  Action Port : ActionPort  ActionType=then
  cfblk11 : Delay
  emi_2046 : Outport
  wires:
  emi_2045/1 -> cfblk11/1
  cfblk11/1 -> emi_2046/1

== system sampleModel7126_pp_1_1/cfblk270/cfblk4 ==
  emi_209 : Inport
  Action Port : ActionPort  ActionType=then
  cfblk4 : simulink/Discrete/Transfer Fcn Lead or Lag  PoleZ=0.95  ZeroZ=0.75  ICPrevOutput=0.0  ICPrevInput=0.0  DoSatur=off
      settings: SourceProductName=Simulink  SourceProductBaseCode=SL
  emi_210 : Outport
  wires:
  emi_209/1 -> cfblk4/1
  cfblk4/1 -> emi_210/1

== system sampleModel7126_pp_1_1/cfblk270/cfblk9 ==
  emi_505 : Inport
  emi_506 : Inport  Port=2
  Action Port : ActionPort  ActionType=then
  cfblk9 : Delay  ShowEnablePort=on
      settings: InputPortMap=u0,e6
  emi_507 : Outport
  wires:
  emi_505/1 -> cfblk9/1
  emi_506/1 -> cfblk9/2
  cfblk9/1 -> emi_507/1

== system sampleModel7126_pp_1_1/cfblk270/emi_2047 ==
  Action Port : ActionPort  ActionType=else
  emi_2048 : Assertion

== system sampleModel7126_pp_1_1/cfblk270/emi_211 ==
  Action Port : ActionPort  ActionType=else
  emi_212 : Assertion

== system sampleModel7126_pp_1_1/cfblk270/emi_508 ==
  Action Port : ActionPort  ActionType=else
  emi_509 : Assertion

== system sampleModel7126_pp_1_1/cfblk271/cfblk10 ==
  emi_1885 : Inport
  Action Port : ActionPort  ActionType=then
  cfblk10 : DiscreteZeroPole  Poles=[0 0.5]  Gain=1  SampleTime=-1
  emi_1886 : Outport
  wires:
  emi_1885/1 -> cfblk10/1
  cfblk10/1 -> emi_1886/1

== system sampleModel7126_pp_1_1/cfblk271/cfblk16 ==
  emi_131 : Inport
  Action Port : ActionPort  ActionType=then
  cfblk16 : Delay
  emi_132 : Outport
  wires:
  emi_131/1 -> cfblk16/1
  cfblk16/1 -> emi_132/1

== system sampleModel7126_pp_1_1/cfblk271/cfblk3 ==
  emi_1913 : Inport
  Action Port : ActionPort  ActionType=then
  cfblk3 : UnitDelay  SampleTime=-1
  emi_1914 : Outport
  wires:
  emi_1913/1 -> cfblk3/1
  cfblk3/1 -> emi_1914/1

== system sampleModel7126_pp_1_1/cfblk271/emi_133 ==
  Action Port : ActionPort  ActionType=else
  emi_134 : Assertion

== system sampleModel7126_pp_1_1/cfblk271/emi_1887 ==
  Action Port : ActionPort  ActionType=else
  emi_1888 : Assertion

== system sampleModel7126_pp_1_1/cfblk271/emi_1915 ==
  Action Port : ActionPort  ActionType=else
  emi_1916 : Assertion

== system sampleModel7126_pp_1_1/cfblk272/cfblk12 ==
  emi_535 : Inport
  Action Port : ActionPort  ActionType=then
  cfblk12 : DataTypeConversion  OutDataTypeStr=double
  emi_536 : Outport
  wires:
  emi_535/1 -> cfblk12/1
  cfblk12/1 -> emi_536/1

== system sampleModel7126_pp_1_1/cfblk272/cfblk4 ==
  emi_1031 : Inport
  Action Port : ActionPort  ActionType=then
  cfblk4 : DiscreteIntegrator  SampleTime=-1  OutDataTypeStr=double  ICPrevOutput=DiscIntNeverNeededParam  ICPrevScaledInput=DiscIntNeverNeededParam
  emi_1032 : Outport
  wires:
  emi_1031/1 -> cfblk4/1
  cfblk4/1 -> emi_1032/1

== system sampleModel7126_pp_1_1/cfblk272/cfblk5 ==
  emi_647 : Inport
  emi_648 : Inport  Port=2
  Action Port : ActionPort  ActionType=then
  cfblk5 : simulink/Continuous/PID Controller (2DOF)  Controller=PID  TimeDomain=Discrete-time  SampleTime=-1  IntegratorMethod=Forward Euler  FilterMethod=Forward Euler  Form=Parallel  UseFilter=on  ControllerParametersSource=internal  P=1  I=1  D=0  N=100  b=1  c=1  InitialConditionSource=internal  InitialConditionForIntegrator=0  InitialConditionForFilter=0  ExternalReset=none  LimitOutput=off  UpperSaturationLimit=inf  LowerSaturationLimit=-inf  LinearizeAsGain=off  AntiWindupMode=none  Kb=1  TrackingMode=off  Kt=1  PParamMin=[]  PParamMax=[]  IParamMin=[]  IParamMax=[]  DParamMin=[]  DParamMax=[]  NParamMin=[]  NParamMax=[]  bParamMin=[]  bParamMax=[]  cParamMin=[]  cParamMax=[]  KbParamMin=[]  KbParamMax=[]  KtParamMin=[]  KtParamMax=[]  POutMin=[]  POutMax=[]  IOutMin=[]  IOutMax=[]  DOutMin=[]  DOutMax=[]  NOutMin=[]  NOutMax=[]  bOutMin=[]  bOutMax=[]  cOutMin=[]  cOutMax=[]  KbOutMin=[]  KbOutMax=[]  KtOutMin=[]  KtOutMax=[]  IntegratorOutMin=[]  IntegratorOutMax=[]  FilterOutMin=[]  FilterOutMax=[]  SumOutMin=[]  SumOutMax=[]  Sum1OutMin=[]  Sum1OutMax=[]  Sum2OutMin=[]  Sum2OutMax=[]  Sum3OutMin=[]  Sum3OutMax=[]  SumI1OutMin=[]  SumI1OutMax=[]  SumI2OutMin=[]  SumI2OutMax=[]  SumI3OutMin=[]  SumI3OutMax=[]  SumDOutMin=[]  SumDOutMax=[]  SaturationOutMin=[]  SaturationOutMax=[]  IntegratorContinuousStateAttributes=''  IntegratorStateMustResolveToSignalObject=off  IntegratorRTWStateStorageClass=Auto  FilterContinuousStateAttributes=''  FilterStateMustResolveToSignalObject=off  FilterRTWStateStorageClass=Auto  DifferentiatorICPrevScaledInput=0  DifferentiatorOutMin=[]  DifferentiatorOutMax=[]  FilterDiffOutCoefMin=[]  FilterDiffOutCoefMax=[]  SumDenOutMin=[]  SumDenOutMax=[]  SumNumOutMin=[]  SumNumOutMax=[]  ReciprocalOutMin=[]  ReciprocalOutMax=[]  DivideOutMin=[]  DivideOutMax=[]  TunerSelectOption=Transfer Function Based (PID Tuner App)
  emi_649 : Outport
  wires:
  emi_647/1 -> cfblk5/1
  emi_648/1 -> cfblk5/2
  cfblk5/1 -> emi_649/1

== system sampleModel7126_pp_1_1/cfblk272/cfblk6 ==
  emi_1454 : Inport
  Action Port : ActionPort  ActionType=then
  cfblk6 : UnitDelay  SampleTime=-1
  emi_1455 : Outport
  wires:
  emi_1454/1 -> cfblk6/1
  cfblk6/1 -> emi_1455/1

== system sampleModel7126_pp_1_1/cfblk272/cfblk7 ==
  emi_846 : Inport
  Action Port : ActionPort  ActionType=then
  cfblk7 : DiscreteTransferFcn
  emi_847 : Outport
  wires:
  emi_846/1 -> cfblk7/1
  cfblk7/1 -> emi_847/1

== system sampleModel7126_pp_1_1/cfblk272/emi_1033 ==
  Action Port : ActionPort  ActionType=else
  emi_1034 : Assertion

== system sampleModel7126_pp_1_1/cfblk272/emi_1456 ==
  Action Port : ActionPort  ActionType=else
  emi_1457 : Assertion

== system sampleModel7126_pp_1_1/cfblk272/emi_537 ==
  Action Port : ActionPort  ActionType=else
  emi_538 : Assertion

== system sampleModel7126_pp_1_1/cfblk272/emi_650 ==
  Action Port : ActionPort  ActionType=else
  emi_651 : Assertion

== system sampleModel7126_pp_1_1/cfblk272/emi_848 ==
  Action Port : ActionPort  ActionType=else
  emi_849 : Assertion

== system sampleModel7126_pp_1_1/cfblk273/cfblk10 ==
  cfblk1 : Inport
  cfblk12 : Inport  Port=2
  Action Port : ActionPort  ActionType=else
  cfblk10 : DiscreteFilter
  cfblk11 : simulink/Continuous/PID Controller  Controller=PID  TimeDomain=Discrete-time  SampleTime=-1  IntegratorMethod=Forward Euler  FilterMethod=Forward Euler  Form=Parallel  UseFilter=on  ControllerParametersSource=internal  P=1  I=1  D=0  N=100  InitialConditionSource=internal  InitialConditionForIntegrator=0  InitialConditionForFilter=0  ExternalReset=none  LimitOutput=off  UpperSaturationLimit=inf  LowerSaturationLimit=-inf  LinearizeAsGain=off  AntiWindupMode=none  Kb=1  TrackingMode=off  Kt=1  PParamMin=[]  PParamMax=[]  IParamMin=[]  IParamMax=[]  DParamMin=[]  DParamMax=[]  NParamMin=[]  NParamMax=[]  KbParamMin=[]  KbParamMax=[]  KtParamMin=[]  KtParamMax=[]  POutMin=[]  POutMax=[]  IOutMin=[]  IOutMax=[]  DOutMin=[]  DOutMax=[]  NOutMin=[]  NOutMax=[]  KbOutMin=[]  KbOutMax=[]  KtOutMin=[]  KtOutMax=[]  IntegratorOutMin=[]  IntegratorOutMax=[]  FilterOutMin=[]  FilterOutMax=[]  SumOutMin=[]  SumOutMax=[]  SumI1OutMin=[]  SumI1OutMax=[]  SumI2OutMin=[]  SumI2OutMax=[]  SumI3OutMin=[]  SumI3OutMax=[]  SumDOutMin=[]  SumDOutMax=[]  SaturationOutMin=[]  SaturationOutMax=[]  IntegratorContinuousStateAttributes=''  IntegratorStateMustResolveToSignalObject=off  IntegratorRTWStateStorageClass=Auto  FilterContinuousStateAttributes=''  FilterStateMustResolveToSignalObject=off  FilterRTWStateStorageClass=Auto  DifferentiatorICPrevScaledInput=0  DifferentiatorOutMin=[]  DifferentiatorOutMax=[]  FilterDiffOutCoefMin=[]  FilterDiffOutCoefMax=[]  SumDenOutMin=[]  SumDenOutMax=[]  SumNumOutMin=[]  SumNumOutMax=[]  ReciprocalOutMin=[]  ReciprocalOutMax=[]  DivideOutMin=[]  DivideOutMax=[]  TunerSelectOption=Transfer Function Based (PID Tuner App)
  cfblk3 : Subsystem  TreatAsAtomicUnit=on
  cfblk4 : Subsystem  TreatAsAtomicUnit=on
  cfblk5 : Subsystem  TreatAsAtomicUnit=on
  cfblk6 : Delay  DelayLengthSource=Input port
      settings: InputPortMap=u0,p1
  cfblk7 : simulink/Discrete/Difference  ICPrevInput=0.0  OutMin=[]  OutMax=[]  OutDataTypeStr=double  OutputDataTypeScalingMode=double  OutDataType=fixdt(1, 16)  OutScaling=2^-10  DoSatur=off
  cfblk8 : DiscreteFir
  cfblk9 : DiscreteFir
  cyemi_{723..732} (10 alike) : DataTypeConversion  OutDataTypeStr=double
  emi_1076 : Subsystem  TreatAsAtomicUnit=on
  emi_1078 : If  IfExpression=0 <= u1  SampleTime=[1 0]
  emi_1079 : DataTypeConversion  OutDataTypeStr=double
  emi_1520 : Subsystem  TreatAsAtomicUnit=on
  emi_1522 : If  IfExpression=-5.427094e-01 <= u1  SampleTime=[1 0]
  emi_1523 : DataTypeConversion  OutDataTypeStr=double
  emi_182 : Subsystem  TreatAsAtomicUnit=on
  emi_184 : If  IfExpression=0 <= u1  SampleTime=[1 0]
  emi_185 : DataTypeConversion  OutDataTypeStr=double
  cfblk2 : Outport
  cfblk13 : Outport  Port=2
  wires:
  cfblk1/1 -> cyemi_727/1, cyemi_729/1
  cfblk7/1 -> cfblk13/1
  cyemi_723/1 -> cfblk10/1
  cfblk9/1 -> cyemi_723/1
  cyemi_724/1 -> cfblk11/1
  cfblk6/1 -> cyemi_724/1
  cfblk12/1 -> cyemi_725/1
  cfblk10/1 -> cyemi_726/1
  cyemi_728/1 -> cfblk6/1
  cyemi_729/1 -> cfblk6/2
  cyemi_730/1 -> cfblk7/1
  cfblk8/1 -> cyemi_730/1, emi_185/1, emi_1079/1
  cyemi_731/1 -> cfblk8/1
  cyemi_732/1 -> cfblk9/1
  cfblk11/1 -> cyemi_732/1
  cyemi_725/1 -> cfblk3/1(emi_180)
  cfblk3/1(emi_181) -> cyemi_728/1, emi_1523/1
  emi_184/1 -> cfblk3/Action
  emi_184/2 -> emi_182/Action
  emi_185/1 -> emi_184/1
  cyemi_727/1 -> cfblk5/1(emi_1074)
  cfblk5/1(emi_1075) -> cyemi_731/1
  emi_1078/1 -> cfblk5/Action
  emi_1078/2 -> emi_1076/Action
  emi_1079/1 -> emi_1078/1
  cyemi_726/1 -> cfblk4/1(emi_1518)
  cfblk4/1(emi_1519) -> cfblk2/1
  emi_1522/1 -> cfblk4/Action
  emi_1522/2 -> emi_1520/Action
  emi_1523/1 -> emi_1522/1

== system sampleModel7126_pp_1_1/cfblk273/cfblk11 ==
  emi_881 : Inport
  Action Port : ActionPort  ActionType=then
  cfblk11 : Delay
  emi_882 : Outport
  wires:
  emi_881/1 -> cfblk11/1
  cfblk11/1 -> emi_882/1

== system sampleModel7126_pp_1_1/cfblk273/cfblk6 ==
  emi_1992 : Inport
  Action Port : ActionPort  ActionType=then
  cfblk6 : DiscreteZeroPole  Poles=[0 0.5]  Gain=1  SampleTime=-1
  emi_1993 : Outport
  wires:
  emi_1992/1 -> cfblk6/1
  cfblk6/1 -> emi_1993/1

== system sampleModel7126_pp_1_1/cfblk273/cfblk9 ==
  cfblk1 : Inport
  cfblk11 : Inport  Port=2
  cfblk12 : Inport  Port=3
  Action Port : ActionPort  ActionType=then
  cfblk10 : DiscreteFilter
  cfblk16 : Subsystem  TreatAsAtomicUnit=on
  cfblk3 : Subsystem  TreatAsAtomicUnit=on
  cfblk4 : DiscreteFilter
  cfblk5 : Subsystem  TreatAsAtomicUnit=on
  cfblk6 : simulink/Discrete/Tapped Delay  vinit=0.0  samptime=-1  NumDelays=1  DelayOrder=Oldest  includeCurrent=off
  cfblk7 : DiscreteStateSpace  SampleTime=-1
  cfblk8 : Subsystem  TreatAsAtomicUnit=on
  cfblk9 : DiscreteFilter
  cyemi_{743..752} (10 alike) : DataTypeConversion  OutDataTypeStr=double
  emi_1005 : Subsystem  TreatAsAtomicUnit=on
  emi_{878,1007,1373,1961} (4 alike) : If  IfExpression=Inf <= u1  SampleTime=[1 0]
  emi_{879,1008,1374,1962} (4 alike) : DataTypeConversion  OutDataTypeStr=double
  emi_1371 : Subsystem  TreatAsAtomicUnit=on
  emi_1959 : Subsystem  TreatAsAtomicUnit=on
  emi_876 : Subsystem  TreatAsAtomicUnit=on
  cfblk2 : Outport
  cfblk13 : Outport  Port=2
  cfblk14 : Outport  Port=3
  cfblk15 : Outport  Port=4
  wires:
  cfblk12/1 -> cfblk2/1
  cfblk10/1 -> cfblk14/1, cfblk13/1, emi_1008/1
  cfblk11/1 -> cyemi_749/1, cyemi_752/1
  cyemi_743/1 -> cfblk10/1
  cfblk4/1 -> cyemi_743/1
  cfblk7/1 -> cyemi_745/1
  cyemi_746/1 -> cfblk4/1
  cfblk6/1 -> cyemi_746/1, emi_879/1, emi_1374/1
  cfblk9/1 -> cyemi_748/1
  cyemi_749/1 -> cfblk6/1
  cyemi_750/1 -> cfblk7/1
  cfblk1/1 -> cyemi_750/1
  cyemi_752/1 -> cfblk9/1
  cyemi_751/1 -> cfblk8/1(emi_874)
  cfblk8/1(emi_875) -> cyemi_744/1
  emi_878/1 -> cfblk8/Action
  emi_878/2 -> emi_876/Action
  emi_879/1 -> emi_878/1
  cyemi_747/1 -> cfblk5/1(emi_1002)
  cyemi_748/1 -> cfblk5/2(emi_1003)
  cfblk5/1(emi_1004) -> cyemi_751/1, emi_1962/1
  emi_1007/1 -> cfblk5/Action
  emi_1007/2 -> emi_1005/Action
  emi_1008/1 -> emi_1007/1
  cyemi_745/1 -> cfblk3/1(emi_1369)
  cfblk3/1(emi_1370) -> cfblk15/1
  emi_1373/1 -> cfblk3/Action
  emi_1373/2 -> emi_1371/Action
  emi_1374/1 -> emi_1373/1
  cyemi_744/1 -> cfblk16/1(emi_1957)
  cfblk16/1(emi_1958) -> cyemi_747/1
  emi_1961/1 -> cfblk16/Action
  emi_1961/2 -> emi_1959/Action
  emi_1962/1 -> emi_1961/1

== system sampleModel7126_pp_1_1/cfblk273/emi_1994 ==
  Action Port : ActionPort  ActionType=else
  emi_1995 : Assertion

== system sampleModel7126_pp_1_1/cfblk273/emi_883 ==
  Action Port : ActionPort  ActionType=else
  emi_884 : Assertion

== system sampleModel7126_pp_1_1/cfblk274/cfblk4 ==
  emi_393 : Inport
  Action Port : ActionPort  ActionType=then
  cfblk4 : DiscreteIntegrator  SampleTime=-1  OutDataTypeStr=double  ICPrevOutput=DiscIntNeverNeededParam  ICPrevScaledInput=DiscIntNeverNeededParam
  emi_394 : Outport
  wires:
  emi_393/1 -> cfblk4/1
  cfblk4/1 -> emi_394/1

== system sampleModel7126_pp_1_1/cfblk274/cfblk5 ==
  emi_1045 : Inport
  Action Port : ActionPort  ActionType=then
  cfblk5 : DiscreteTransferFcn
  emi_1046 : Outport
  wires:
  emi_1045/1 -> cfblk5/1
  cfblk5/1 -> emi_1046/1

== system sampleModel7126_pp_1_1/cfblk274/cfblk6 ==
  emi_888 : Inport
  emi_889 : Inport  Port=2
  Action Port : ActionPort  ActionType=then
  cfblk6 : Delay  ShowEnablePort=on
      settings: InputPortMap=u0,e6
  emi_890 : Outport
  wires:
  emi_888/1 -> cfblk6/1
  emi_889/1 -> cfblk6/2
  cfblk6/1 -> emi_890/1

== system sampleModel7126_pp_1_1/cfblk274/cfblk7 ==
  emi_2094 : Inport
  emi_2095 : Inport  Port=2
  Action Port : ActionPort  ActionType=then
  cfblk7 : Delay  ShowEnablePort=on
      settings: InputPortMap=u0,e6
  emi_2096 : Outport
  wires:
  emi_2094/1 -> cfblk7/1
  emi_2095/1 -> cfblk7/2
  cfblk7/1 -> emi_2096/1

== system sampleModel7126_pp_1_1/cfblk274/emi_1047 ==
  Action Port : ActionPort  ActionType=else
  emi_1048 : Assertion

== system sampleModel7126_pp_1_1/cfblk274/emi_2097 ==
  Action Port : ActionPort  ActionType=else
  emi_2098 : Assertion

== system sampleModel7126_pp_1_1/cfblk274/emi_395 ==
  Action Port : ActionPort  ActionType=else
  emi_396 : Assertion

== system sampleModel7126_pp_1_1/cfblk274/emi_891 ==
  Action Port : ActionPort  ActionType=else
  emi_892 : Assertion
